simulink model "billiard"  (R2019a)
settings: Solver=VariableStepAuto  StartTime=0.0  StopTime=10.0  RelTol=1e-3
model workspace (MAT data in the model file):
  yvelov = Simulink.NumericType
  yvelov.DataTypeMode = 'Double'
  yvelov.SignednessBool = 1
  yvelov.WordLength = 64
  yvelov.FixedExponent = 0
  yvelov.SlopeAdjustmentFactor = 1
  yvelov.Bias = 0
  yvelov.DataTypeOverride = 'Inherit'
  yvelov.IsAlias = 0
  yvelov.DataScope = 'Auto'
settings Model: Creator=kejo5874  LastModifiedBy=kejo5874

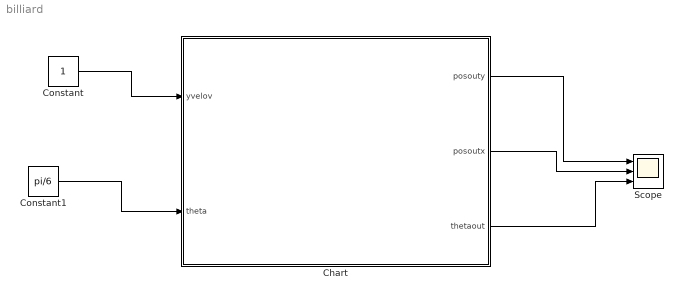
== system billiard ==
  Chart : Stateflow chart  BlockKeywords=__PRM__SERIALIZED__DATA__:Stateflow Chart,Stateflow Diagram  TreatAsAtomicUnit=on
  Constant : Constant
  Constant1 : Constant  Value=pi/6
  Scope : Scope  NumInputPorts=3
  wires:
  Constant/1 -> Chart/1(yvelov)
  Chart/1(posouty) -> Scope/1
  Chart/2(posoutx) -> Scope/2
  Chart/3(thetaout) -> Scope/3
  Constant1/1 -> Chart/2(theta)

== stateflow chart billiard/Chart ==
  state Ball
    du:
    posy_dot = yVelocity;
    posx_dot = xVelocity;
    posouty = posy;
    posoutx = posx;
    thetaout = theta;
  (default) -> Ball : {
      | posx = 1;
      | posy = 0;
      | yvelo = velomag*sin(pi/6);
      | xvelo = velomag*cos(pi/6);
      | }
  Ball -> Ball [order 1] : [posx <= 0 || posx >= 2]{xvelo = -xvelo}
  Ball -> Ball [order 2] : [posy<= 0 || posy >= 1]{yvelo = -yvelo}
  data: posx local; posy local; yVelocity constant double; posouty output; posoutx output; thetaout output; posy_dot local; posx_dot local; xVelocity constant double; xvelo local; yvelo local; yvelov input; velomag constant double; theta input
